simulink model "Complete_plant"  (R2024b)
settings: Solver=VariableStepAuto  StartTime=0.0  StopTime=simt  RelTol=1e-3
undefined symbols (not defined in the file): Kd, Ki, Kp, T, theta
settings Model: Creator=crunc  LastModifiedBy=crunc

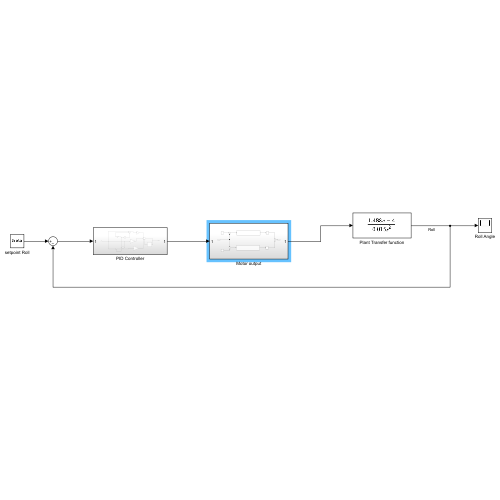
[thumbnail: Simulink's stored preview of the top-level diagram]
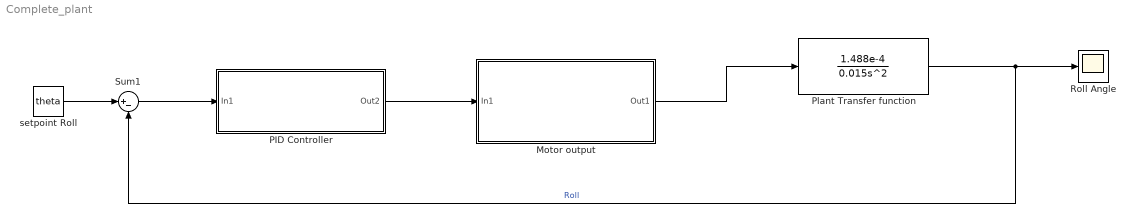
== system Complete_plant ==
  Motor output : Subsystem
  PID Controller : Subsystem
  Plant Transfer function : TransferFcn  Numerator=[1.488e-4]  Denominator=[0.015 0 0]
  Roll Angle : Scope
  Sum1 : Sum  Inputs=|+-
  setpoint Roll : Constant  Value=theta
  wires:
  Motor output/1(Out1) -> Plant Transfer function/1
  setpoint Roll/1 -> Sum1/1
  Plant Transfer function/1 -> Roll Angle/1, Sum1/2  "Roll"
  Sum1/1 -> PID Controller/1(In1)
  PID Controller/1(Out2) -> Motor output/1(In1)

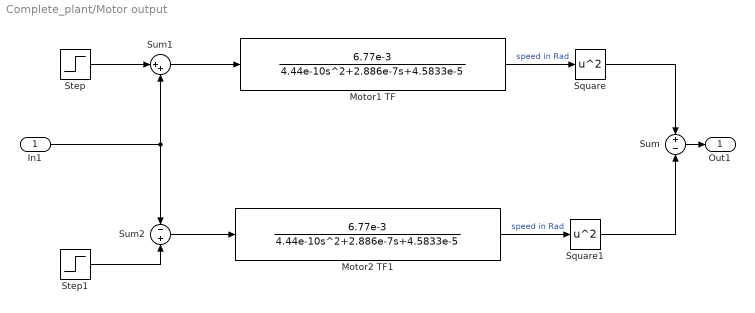
== system Complete_plant/Motor output ==
  In1 : Inport
  " Motor1 TF" : TransferFcn  Numerator=[6.77e-3]  Denominator=[4.44e-10 2.886e-7 4.5833e-5]
  " Motor2 TF1" : TransferFcn  Numerator=[6.77e-3]  Denominator=[4.44e-10 2.886e-7 4.5833e-5]
  Square : Math  Operator=square
  Square1 : Math  Operator=square
  Step : Step  SampleTime=0
  Step1 : Step  SampleTime=0
  Sum : Sum  Inputs=+-
  Sum1 : Sum  Inputs=|++
  Sum2 : Sum  Inputs=-+
  Out1 : Outport
  wires:
  Square1/1 -> Sum/2
  In1/1 -> Sum1/2, Sum2/1
  " Motor2 TF1"/1 -> Square1/1  "speed in Rad"
  Step/1 -> Sum1/1
  " Motor1 TF"/1 -> Square/1  "speed in Rad"
  Square/1 -> Sum/1
  Step1/1 -> Sum2/2
  Sum/1 -> Out1/1
  Sum1/1 -> " Motor1 TF"/1
  Sum2/1 -> " Motor2 TF1"/1

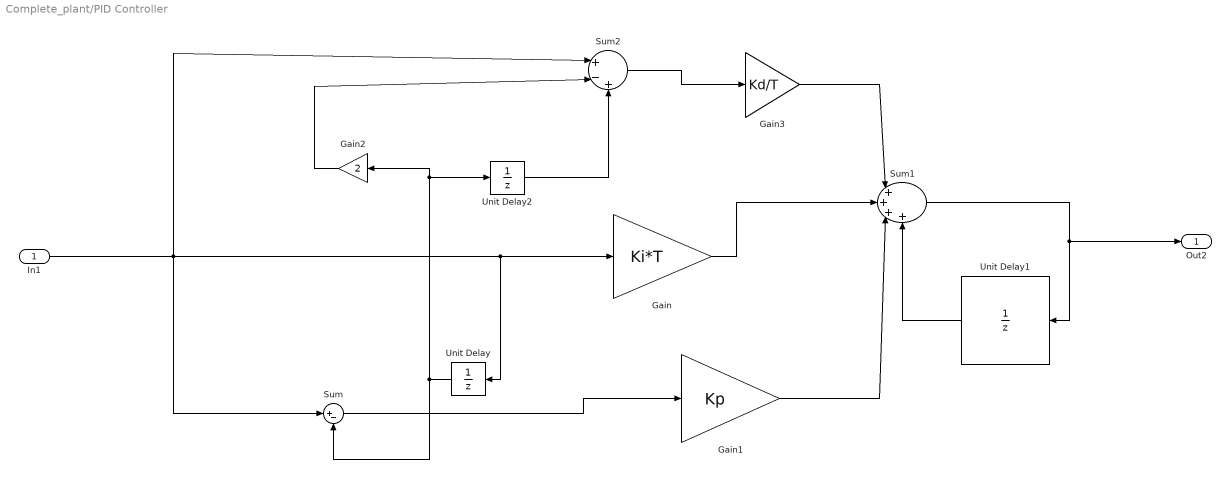
== system Complete_plant/PID Controller ==
  In1 : Inport
  Gain : Gain  Gain=Ki*T
  Gain1 : Gain  Gain=Kp
  Gain2 : Gain  Gain=2
  Gain3 : Gain  Gain=Kd/T
  Sum : Sum  Inputs=|+-
  Sum1 : Sum  Inputs=|++++
  Sum2 : Sum  Inputs=|+-+
  Unit Delay : UnitDelay  SampleTime=-1  HasFrameUpgradeWarning=on
  Unit Delay1 : UnitDelay  SampleTime=-1  HasFrameUpgradeWarning=on
  Unit Delay2 : UnitDelay  SampleTime=-1  HasFrameUpgradeWarning=on
  Out2 : Outport
  wires:
  Unit Delay1/1 -> Sum1/4
  Gain1/1 -> Sum1/3
  In1/1 -> Sum2/1, Sum/1, Unit Delay/1, Gain/1
  Gain/1 -> Sum1/2
  Unit Delay/1 -> Unit Delay2/1, Gain2/1, Sum/2
  Sum1/1 -> Unit Delay1/1, Out2/1
  Sum/1 -> Gain1/1
  Gain2/1 -> Sum2/2
  Unit Delay2/1 -> Sum2/3
  Sum2/1 -> Gain3/1
  Gain3/1 -> Sum1/1
